simulink model "Sim_VSI_Resonant"  (R2025b)
settings: Solver=VariableStepAuto  StartTime=0.0  StopTime=0.3  FixedStep=Ts  RelTol=1e-3
values from neighbouring files (symbols this model uses):
  A_gamma = [-Rfp/Lfp  0           1/Lfp ... (first row only)    [Variables.m]
  Ard = blkdiag(Ard1,Ard3,Ard5,Ard7)    [Init_Gamma_Resonant.m]    (also in LQR_Search.m = [])
  B_gamma = [1/Lfp; 0; 0]    [Variables.m]
  Brd = [Brd1;Brd3;Brd5;Brd7]    [Init_Gamma_Resonant.m]    (also in LQR_Search.m = [])
  C_gamma = eye(3)    [Variables.m]
  Ha = [0 0 1 0 0 0 0 0 0 0 ... (first row only)    [HDT_Unified_Init.m]    (also in Init_Gamma_Resonant.m = [1 0 0])
  Kr = []    [Final_Value.m]    (also in LQR_Search.m = zeros(size(K,1),0))
  Ku = K(:, nx+1 : nx+nu)    [Final_Value.m]    (also in LQR_Search.m = K(:,idx_x_end+1:idx_u_end))
  Kx = K(:, 1:nx)    [Final_Value.m]    (also in LQR_Search.m = K(:,1:idx_x_end))
  Ts = 1/(2*fsw)    (= 2.5e-05)    [Variables.m]    (also in Variables_HDT.m)
  w = 2*pi*50    (= 314.159265359)    [Variables.m]    (also in Variables_HDT.m)
settings Model: Creator=dfigueroa  LastModifiedBy=dfigueroa

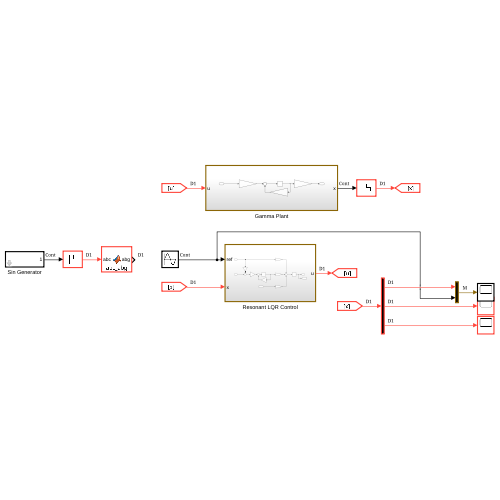
[thumbnail: Simulink's stored preview of the top-level diagram]
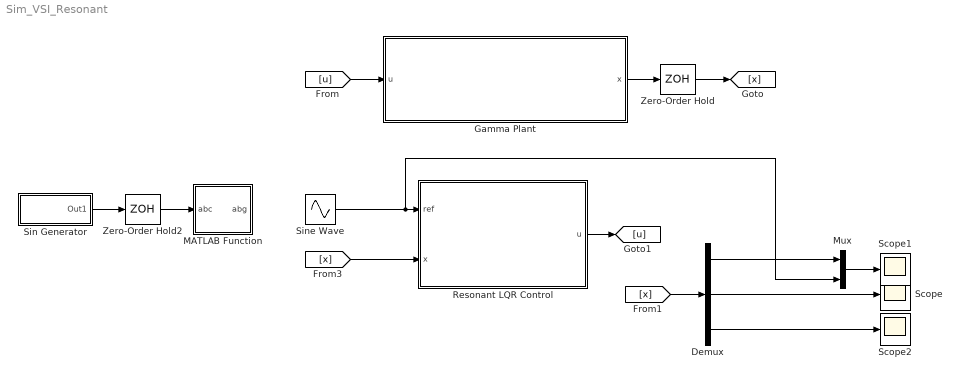
== system Sim_VSI_Resonant ==
  Demux : Demux  Outputs=3
  Gamma Plant : Subsystem
  MATLAB Function : MATLAB Function  TreatAsAtomicUnit=on
  Mux : Mux  Inputs=2
  Resonant LQR Control : Subsystem
  Scope : Scope
      settings: ActiveDisplayYMinimum=-80.048593068021944  ActiveDisplayYMaximum=89.806775781162116
  Scope1 : Scope
      settings: ActiveDisplayYMinimum=-6.25  ActiveDisplayYMaximum=6.25
  Scope2 : Scope
      settings: ActiveDisplayYMinimum=-80.048593068021944  ActiveDisplayYMaximum=89.806775781162116  DataLoggingVariableName=ScopeData2
  Sin Generator : Subsystem  mask{w=w, Amp=5, Tset=0.02, Tstep=0}
      mask prompts: w "Frequency"; Amp "Reference Amplitude"; Tset "Set Time [s]"; Tstep "Step Time"
  Sine Wave : Sin  Amplitude=5  Frequency=100*pi  SampleTime=0
  Zero-Order Hold : ZeroOrderHold  SampleTime=Ts
  Zero-Order Hold2 : ZeroOrderHold  SampleTime=Ts
  wires:
  Demux/2 -> Scope/1
  [x] -> Demux/1
  Zero-Order Hold/1 -> [x]
  Zero-Order Hold2/1 -> MATLAB Function/1(abc)
  Gamma Plant/1(x) -> Zero-Order Hold/1
  [u] -> Gamma Plant/1(u)
  [x] -> Resonant LQR Control/2(x)
  Resonant LQR Control/1(u) -> [u]
  Sin Generator/1(Out1) -> Zero-Order Hold2/1
  Demux/1 -> Mux/1
  Demux/3 -> Scope2/1
  Sine Wave/1 -> Mux/2, Resonant LQR Control/1(ref)
  Mux/1 -> Scope1/1

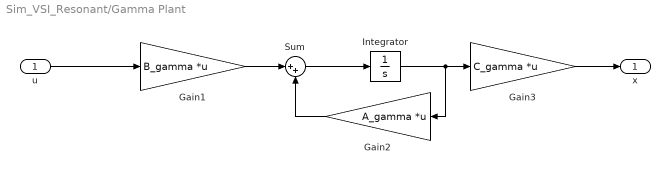
== system Sim_VSI_Resonant/Gamma Plant ==
  u : Inport
  Gain1 : Gain  Gain=B_gamma  Multiplication=Matrix(K*u)
  Gain2 : Gain  Gain=A_gamma  Multiplication=Matrix(K*u)
  Gain3 : Gain  Gain=C_gamma  Multiplication=Matrix(K*u)
  Integrator : Integrator
  Sum : Sum  Inputs=|++
  x : Outport
  wires:
  u/1 -> Gain1/1
  Gain2/1 -> Sum/2
  Sum/1 -> Integrator/1
  Integrator/1 -> Gain3/1, Gain2/1
  Gain1/1 -> Sum/1
  Gain3/1 -> x/1

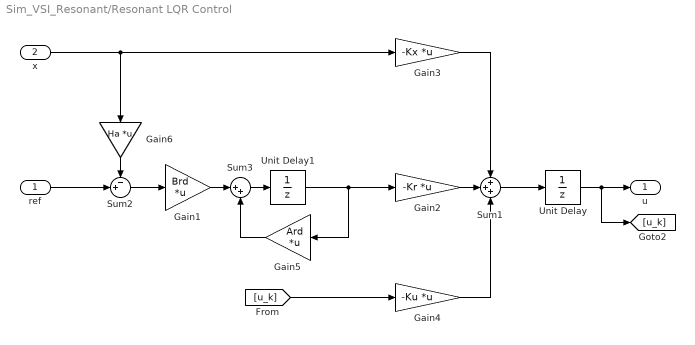
== system Sim_VSI_Resonant/Resonant LQR Control ==
  ref : Inport
  x : Inport  Port=2
  Gain1 : Gain  Gain=Brd  Multiplication=Matrix(K*u)
  Gain2 : Gain  Gain=-Kr  Multiplication=Matrix(K*u)
  Gain3 : Gain  Gain=-Kx  Multiplication=Matrix(K*u)
  Gain4 : Gain  Gain=-Ku  Multiplication=Matrix(K*u)
  Gain5 : Gain  Gain=Ard  Multiplication=Matrix(K*u)
  Gain6 : Gain  Gain=Ha  Multiplication=Matrix(K*u)
  Sum1 : Sum  Inputs=+++
  Sum2 : Sum  Inputs=-+|
  Sum3 : Sum  Inputs=|++
  Unit Delay : UnitDelay  SampleTime=Ts  HasFrameUpgradeWarning=on
  Unit Delay1 : UnitDelay  SampleTime=Ts  HasFrameUpgradeWarning=on
  u : Outport
  wires:
  x/1 -> Gain6/1, Gain3/1
  Gain6/1 -> Sum2/1
  Unit Delay/1 -> [u_k], u/1
  ref/1 -> Sum2/2
  Gain2/1 -> Sum1/2
  Gain3/1 -> Sum1/1
  Gain4/1 -> Sum1/3
  [u_k] -> Gain4/1
  Sum1/1 -> Unit Delay/1
  Sum2/1 -> Gain1/1
  Gain1/1 -> Sum3/1
  Sum3/1 -> Unit Delay1/1
  Gain5/1 -> Sum3/2
  Unit Delay1/1 -> Gain5/1, Gain2/1

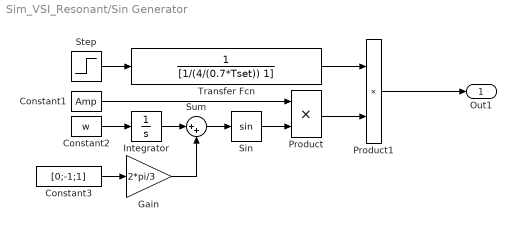
== system Sim_VSI_Resonant/Sin Generator ==
  Constant1 : Constant  Value=Amp
  Constant2 : Constant  Value=w
  Constant3 : Constant  Value=[0;-1;1]
  Gain : Gain  Gain=2*pi/3
  Integrator : Integrator
  Product : Product
  Product1 : Product
  Sin : Trigonometry
  Step : Step  Time=Tstep  SampleTime=0
  Sum : Sum  Inputs=|++
  Transfer Fcn : TransferFcn  Denominator=[1/(4/(0.7*Tset)) 1]
  Out1 : Outport
  wires:
  Sum/1 -> Sin/1
  Transfer Fcn/1 -> Product1/1
  Constant2/1 -> Integrator/1
  Integrator/1 -> Sum/1
  Constant1/1 -> Product/1
  Constant3/1 -> Gain/1
  Product1/1 -> Out1/1
  Gain/1 -> Sum/2
  Step/1 -> Transfer Fcn/1
  Sin/1 -> Product/2
  Product/1 -> Product1/2

== matlab function Sim_VSI_Resonant/MATLAB Function ==
  data: abc input; abg output
function abg = abc_abg(abc)
    a = abc(1);
    b = abc(2);
    c = abc(3);

    alpha = (2*a - b - c)/3;
    beta  = (b - c)/sqrt(3);
    gamma = (a + b + c)/3;

    abg = [alpha; beta; gamma];
end
